simulink model "GA_PSCAV"  (R2019a)
settings: Solver=VariableStepAuto  StartTime=0.0  StopTime=0.8  RelTol=1e-3
libraries: powerlib x12, re_lib x3, simulink x1
settings Model: Creator=user  LastModifiedBy=engma

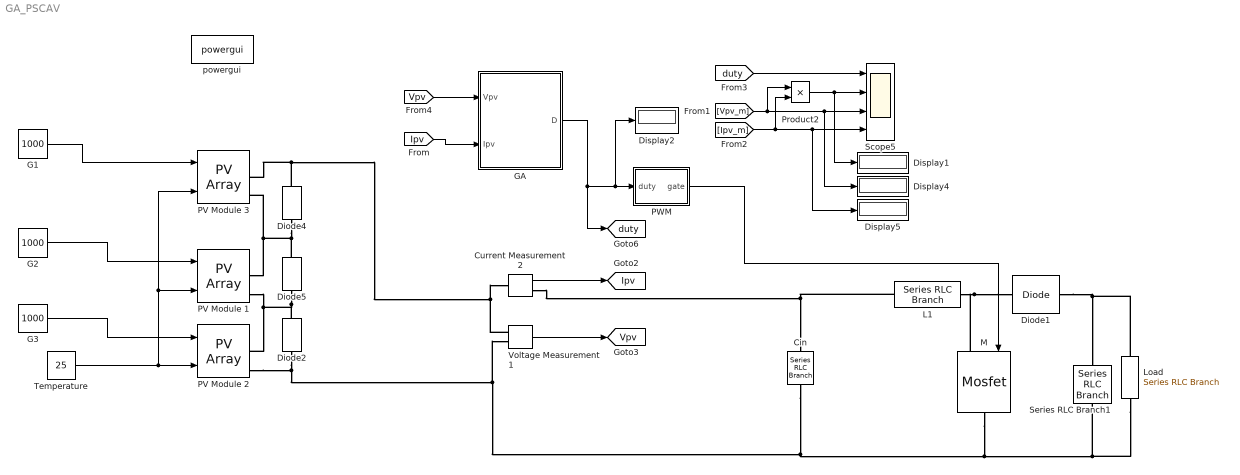
== system GA_PSCAV ==
  Cin : powerlib/Elements/Series RLC Branch  LConnTagsString=__new0  RConnTagsString=__new0  BranchType=C  Resistance=1e-3  Inductance=250e-6  SetiL0=off  InitialCurrent=0  Capacitance=10e-2  Setx0=off  InitialVoltage=0  Measurements=None
      settings: SourceProductName=Simscape Electrical
  Current Measurement2 : powerlib/Measurements/Current Measurement  PhasorSimulation=off  OutputType=Complex  PSBequivalent=0
      settings: SourceProductName=Simscape Electrical
  Diode1 : powerlib/Power Electronics/Diode  Ron=1e-3  Lon=0  Vf=0  IC=0  UseSnubber=off  Rs=inf  Cs=inf  Measurements=off
      settings: SourceProductName=Simscape Electrical
  Diode2 : powerlib/Power Electronics/Diode  Ron=0.001  Lon=0  Vf=0.5  IC=0  UseSnubber=off  Rs=500  Cs=250e-9  Measurements=off
      settings: SourceProductName=Simscape Electrical
  Diode4 : powerlib/Power Electronics/Diode  Ron=0.001  Lon=0  Vf=0.5  IC=0  UseSnubber=off  Rs=500  Cs=250e-9  Measurements=off
      settings: SourceProductName=Simscape Electrical
  Diode5 : powerlib/Power Electronics/Diode  Ron=0.001  Lon=0  Vf=0.5  IC=0  UseSnubber=off  Rs=500  Cs=250e-9  Measurements=off
      settings: SourceProductName=Simscape Electrical
  Display{1..2,4..5} (4 alike) : Display
  G1 : Constant  Value=1000
  G2 : Constant  Value=1000
  G3 : Constant  Value=1000
  "GA " : MATLAB Function  TreatAsAtomicUnit=on
  L1 : powerlib/Elements/Series RLC Branch  LConnTagsString=__new0  RConnTagsString=__new0  BranchType=L  Resistance=1e-3  Inductance=5e-6  SetiL0=off  InitialCurrent=0  Capacitance=1e-6  Setx0=off  InitialVoltage=0  Measurements=None
      settings: SourceProductName=Simscape Electrical
  Load : powerlib/Elements/Series RLC Branch  LConnTagsString=__new0  RConnTagsString=__new0  BranchType=R  Resistance=100  Inductance=1e-3  SetiL0=off  InitialCurrent=0  Capacitance=1e-6  Setx0=off  InitialVoltage=0  Measurements=None
      settings: SourceProductName=Simscape Electrical
  M : powerlib/Power Electronics/Mosfet  Ron=1e-3  Lon=0  Rd=1e-3  Vfd=0  IC=0  Rs=1e5  Cs=inf  Measurements=off
      settings: SourceProductName=Simscape Electrical
  PV Module 1 : re_lib/Solar/PV Array  Npar=1  Nser=1  PlotType=array @ 1000 W/m2 & specified temperatures  S_vec="[ 1000  500  100 ]"  Temp_C_vec="[ 45 25  ]"  ModuleName=Kyocera Solar KD320GX-LPB  PlotWhenSelected=off  Pm=320.399  Ncell=80  Voc=49.5  Isc=8.6  Vm=40.1  Im=7.99  beta_Voc_pc=-0.37  alpha_Isc_pc=0.041  beta_Voc=-0.18315  alpha_Isc=0.003526  IL=8.6148  I0=3.9672e-10  nI=1.0129  Rsh=238.5428  Rs=0.40954  BAL=off  Tc=1e-6  Tfilter=1e-4
      settings: SourceProductName=Simscape Electrical
  PV Module 2 : re_lib/Solar/PV Array  Npar=1  Nser=1  PlotType=array @ 1000 W/m2 & specified temperatures  S_vec="[ 1000  500  100 ]"  Temp_C_vec="[ 45 25  ]"  ModuleName=Kyocera Solar KD320GX-LPB  PlotWhenSelected=off  Pm=320.399  Ncell=80  Voc=49.5  Isc=8.6  Vm=40.1  Im=7.99  beta_Voc_pc=-0.37  alpha_Isc_pc=0.041  beta_Voc=-0.18315  alpha_Isc=0.003526  IL=8.6148  I0=3.9672e-10  nI=1.0129  Rsh=238.5428  Rs=0.40954  BAL=off  Tc=1e-6  Tfilter=1e-4
      settings: SourceProductName=Simscape Electrical
  PV Module 3 : re_lib/Solar/PV Array  Npar=1  Nser=1  PlotType=array @ 1000 W/m2 & specified temperatures  S_vec="[ 1000  500  100 ]"  Temp_C_vec="[ 45 25  ]"  ModuleName=Kyocera Solar KD320GX-LPB  PlotWhenSelected=off  Pm=320.399  Ncell=80  Voc=49.5  Isc=8.6  Vm=40.1  Im=7.99  beta_Voc_pc=-0.37  alpha_Isc_pc=0.041  beta_Voc=-0.18315  alpha_Isc=0.003526  IL=8.6148  I0=3.9672e-10  nI=1.0129  Rsh=238.5428  Rs=0.40954  BAL=off  Tc=1e-6  Tfilter=1e-4
      settings: SourceProductName=Simscape Electrical
  PWM : Subsystem
  Product2 : Product
  Scope5 : Scope  NumInputPorts=4
  Series RLC Branch1 : powerlib/Elements/Series RLC Branch  LConnTagsString=__new0  RConnTagsString=__new0  BranchType=C  Resistance=1e-4  Inductance=200e-6  SetiL0=off  InitialCurrent=0  Capacitance=75e-5  Setx0=off  InitialVoltage=40  Measurements=None
      settings: SourceProductName=Simscape Electrical
  Temperature : Constant  Value=25
  Voltage Measurement1 : powerlib/Measurements/Voltage Measurement  PhasorSimulation=off  OutputType=Complex  PSBequivalent=0
      settings: SourceProductName=Simscape Electrical
  powergui : powerlib/powergui  Priority=1  SimulationMode=Discrete  SampleTime=1e-6  frequency=60  Iterations=50  frequencyindice=0  Pbase=100e6  ErrMax=1e-4  UnitsV=kV  UnitsW=MW  buscounter=0  FunctionMessages=off  echomessages=off  EnableUseOfTLC=off  CurrentSourceSwitches=off  DisableSnubberDevices=off  DisableRonSwitches=off  DisableVfSwitches=off  DisplayEquations=off  AutomaticDiscreteSolvers=off  SolverType=Backward Euler  Interpol=off  ExternalGateDelay=off  methode=off  Ts=0  x0status=blocks  SPID=on  SwTol=0  HookPort=off  NonlinearTolerance=1e-4  nMaxIteration=100  ContinueOnMaxIteration=off  RestoreLinks=warning  ResistiveCurrentMeasurement=off  Frange=[0:2:500]  Ylog=off  Xlog=on  ShowGrid=off  save=off  variable=ZData  structure=0  ZoomFFT=off  StartTime=0.0  cycles=1  DisplayStyle=1  fundamental=60  FreqAxis=off  MaxFrequency=1000  frequencyindicesteady=1  RmsSteady=1  display=off
      settings: SourceProductName=Simscape Electrical
  tag scope: Ipv=global, Vpv=global, duty=global
  wires:
  PWM/1(gate) -> M/1
  Temperature/1 -> PV Module 2/2, PV Module 1/2, PV Module 3/2
  [Vpv] -> "GA "/1(Vpv)
  G1/1 -> PV Module 3/1
  G3/1 -> PV Module 2/1
  "GA "/1(D) -> [duty], Display2/1, PWM/1(duty)
  Voltage Measurement1/1 -> [Vpv]
  Product2/1 -> Display1/1, Scope5/2
  [duty] -> Scope5/1
  [Vpv_m] -> Product2/1, Display4/1, Scope5/3
  G2/1 -> PV Module 1/1
  Current Measurement2/1 -> [Ipv]
  [Ipv_m] -> Product2/2, Display5/1, Scope5/4
  [Ipv] -> "GA "/2(Ipv)
  connections:
  Diode1/LConn1 -- M/LConn1 -- L1/RConn1
  Diode4/RConn1 -- PV Module 3/RConn1 -- Voltage Measurement1/LConn1 -- Current Measurement2/LConn1
  PV Module 3/RConn2 -- Diode4/LConn1 -- Diode5/RConn1 -- PV Module 1/RConn1
  L1/LConn1 -- Current Measurement2/RConn1 -- Cin/LConn1
  PV Module 1/RConn2 -- PV Module 2/RConn1 -- Diode2/RConn1 -- Diode5/LConn1
  Diode1/RConn1 -- Load/LConn1 -- Series RLC Branch1/LConn1
  M/RConn1 -- Voltage Measurement1/LConn2 -- Diode2/LConn1 -- PV Module 2/RConn2 -- Cin/RConn1 -- Load/RConn1 -- Series RLC Branch1/RConn1

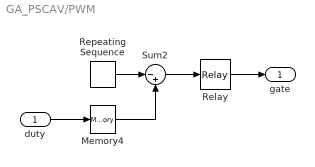
== system GA_PSCAV/PWM ==
  duty : Inport
  Memory4 : Memory
  Relay : Relay
  Repeating Sequence : simulink/Sources/Repeating Sequence  rep_seq_t=[0 1/25000]  rep_seq_y=[0 1]
  Sum2 : Sum  Inputs=|-+
  gate : Outport  VectorParamsAs1DForOutWhenUnconnected=on
  wires:
  Relay/1 -> gate/1
  Repeating Sequence/1 -> Sum2/1
  Sum2/1 -> Relay/1
  Memory4/1 -> Sum2/2
  duty/1 -> Memory4/1

== matlab function GA_PSCAV/GA  ==
  settings: updateMethod=DISCRETE  sampleTime=1e-4
  data: Vpv input; D output; Ipv input
function D = GA(Vpv,Ipv)
D=100.78;

end
